simulink model "scattering_based_bi_teleop_pf2"  (R2020b)
settings: Solver=VariableStepAuto  StartTime=0.0  StopTime=4.0  RelTol=1e-3
values from neighbouring files (symbols this model uses):
  A = 1    [four_channel_bilateral_teleoperation_kalman_params.m]    (also in four_channel_bilateral_teleoperation_params.m; kalman_test.m = [1 Ts Ts^2/2; 0 1 Ts; 0 0 1]; recursive_estimation.m = [1 Ts Ts^2/2; 0 1 Ts; 0 0 1]; scattering_based_bi_teleop_pf_kalman_params.m)
  b = 1    [scattering_based_bi_teleop_pf_kalman_params.m]    (also in scattering_based_bi_teleop_pf_params.m; scattering_based_bi_teleop_pp_kalman_params.m; scattering_based_bi_teleop_pp_params.m = 0.9; scattering_based_bilateral_teleoperation_pp_params.m = 0.234)
  Be = 100    [four_channel_bilateral_teleoperation_architecture_params.m]    (also in four_channel_bilateral_teleoperation_kalman_params.m = 0; four_channel_bilateral_teleoperation_params.m = 0; scattering_based_bi_teleop_pf_kalman_params.m = 10; scattering_based_bi_teleop_pf_params.m = 10)
  Bh = 70    [four_channel_bilateral_teleoperation_architecture_params.m]    (also in four_channel_bilateral_teleoperation_kalman_params.m; four_channel_bilateral_teleoperation_params.m; scattering_based_bi_teleop_pf_kalman_params.m = 1.5; scattering_based_bi_teleop_pf_params.m = 1.5)
  Bm = 1    [four_channel_bilateral_teleoperation_architecture_params.m]    (also in four_channel_bilateral_teleoperation_kalman_params.m = 0.8; four_channel_bilateral_teleoperation_params.m = 0.8; scattering_based_bi_teleop_pf_kalman_params.m = 0; scattering_based_bi_teleop_pf_params.m = 0)
  Bs = 1    [four_channel_bilateral_teleoperation_architecture_params.m]    (also in four_channel_bilateral_teleoperation_kalman_params.m = 3.2; four_channel_bilateral_teleoperation_params.m = 3.2; scattering_based_bi_teleop_pf_kalman_params.m = 40; scattering_based_bi_teleop_pf_params.m = 3)
  delay = 10    [scattering_based_bi_teleop_pf_kalman_params.m]    (also in scattering_based_bi_teleop_pf_params.m = 1; scattering_based_bi_teleop_pp_kalman_params.m = 1; scattering_based_bi_teleop_pp_params.m = 1; tank_based_bi_teleop_pf_kalman.m)
  Dh = 500    [four_channel_bilateral_teleoperation_kalman_params.m]    (also in four_channel_bilateral_teleoperation_params.m; scattering_based_bi_teleop_pf_kalman_params.m = 0; scattering_based_bi_teleop_pf_params.m = 17; scattering_based_bi_teleop_pp_kalman_params.m = 0)
  Dm = 5    [four_channel_bilateral_teleoperation_architecture_params.m]    (also in four_channel_bilateral_teleoperation_kalman_params.m = 0; four_channel_bilateral_teleoperation_params.m = 0; scattering_based_bi_teleop_pf_kalman_params.m = 0; scattering_based_bi_teleop_pf_params.m = 0)
  Ds = 10    [four_channel_bilateral_teleoperation_architecture_params.m]    (also in four_channel_bilateral_teleoperation_kalman_params.m = 0; four_channel_bilateral_teleoperation_params.m = 0; scattering_based_bi_teleop_pf_kalman_params.m = 0; scattering_based_bi_teleop_pf_params.m = 0)
  Fc = 1    [four_channel_bilateral_teleoperation_kalman_params.m]    (also in four_channel_bilateral_teleoperation_params.m; kalman_test.m = 10; scattering_based_bi_teleop_pf_kalman_params.m = 0.1; scattering_based_bi_teleop_pf_params.m)
  Filter = 8    [scattering_based_bi_teleop_pf_kalman_params.m]    (also in scattering_based_bi_teleop_pf_params.m = 100; scattering_based_bi_teleop_pp_kalman_params.m = 10; scattering_based_bi_teleop_pp_params.m = 5; tank_based_bi_teleop_pf_kalman.m = 100)
  Fip = 1    [four_channel_bilateral_teleoperation_kalman_params.m]    (also in four_channel_bilateral_teleoperation_params.m; scattering_based_bi_teleop_pf_kalman_params.m = 5; scattering_based_bi_teleop_pf_params.m = 10; scattering_based_bi_teleop_pp_kalman_params.m = 5)
  Je = 0    [four_channel_bilateral_teleoperation_architecture_params.m]    (also in four_channel_bilateral_teleoperation_kalman_params.m; four_channel_bilateral_teleoperation_params.m; scattering_based_bi_teleop_pf_kalman_params.m; scattering_based_bi_teleop_pf_params.m)
  Jh = 0.5    [four_channel_bilateral_teleoperation_architecture_params.m]    (also in four_channel_bilateral_teleoperation_kalman_params.m; four_channel_bilateral_teleoperation_params.m; scattering_based_bi_teleop_pf_kalman_params.m = 0; scattering_based_bi_teleop_pf_params.m = 0.05)
  Ke = 200    [four_channel_bilateral_teleoperation_architecture_params.m]    (also in four_channel_bilateral_teleoperation_kalman_params.m = 50; four_channel_bilateral_teleoperation_params.m = 50; scattering_based_bi_teleop_pf_kalman_params.m; scattering_based_bi_teleop_pf_params.m)
  Kh = 2000    [four_channel_bilateral_teleoperation_architecture_params.m]    (also in four_channel_bilateral_teleoperation_kalman_params.m; four_channel_bilateral_teleoperation_params.m; scattering_based_bi_teleop_pf_kalman_params.m = 1; scattering_based_bi_teleop_pf_params.m = 0)
  Km = 1    [four_channel_bilateral_teleoperation_architecture_params.m]    (also in four_channel_bilateral_teleoperation_kalman_params.m; four_channel_bilateral_teleoperation_params.m; scattering_based_bi_teleop_pf_kalman_params.m = 0; scattering_based_bi_teleop_pf_params.m = 0)
  Ks = 1    [four_channel_bilateral_teleoperation_architecture_params.m]    (also in four_channel_bilateral_teleoperation_kalman_params.m = 4; four_channel_bilateral_teleoperation_params.m = 4; scattering_based_bi_teleop_pf_kalman_params.m = 50; scattering_based_bi_teleop_pf_params.m = 110)
  Mm = 0.5    [four_channel_bilateral_teleoperation_architecture_params.m]    (also in four_channel_bilateral_teleoperation_kalman_params.m; four_channel_bilateral_teleoperation_params.m; scattering_based_bi_teleop_pf_kalman_params.m; scattering_based_bi_teleop_pf_params.m)
  Ms = 2    [four_channel_bilateral_teleoperation_architecture_params.m]    (also in four_channel_bilateral_teleoperation_kalman_params.m; four_channel_bilateral_teleoperation_params.m; scattering_based_bi_teleop_pf_kalman_params.m; scattering_based_bi_teleop_pf_params.m)
  Ph = 2000    [four_channel_bilateral_teleoperation_kalman_params.m]    (also in four_channel_bilateral_teleoperation_params.m = 50500; scattering_based_bi_teleop_pf_kalman_params.m = 5; scattering_based_bi_teleop_pf_params.m = 23; scattering_based_bi_teleop_pp_kalman_params.m = 6)
  Ts = 0.001    [four_channel_bilateral_teleoperation_kalman_params.m]    (also in four_channel_bilateral_teleoperation_params.m; kalman_test.m; recursive_estimation.m; scattering_based_bi_teleop_pf_kalman_params.m)
settings Model: Creator=anuj  LastModifiedBy=filippo

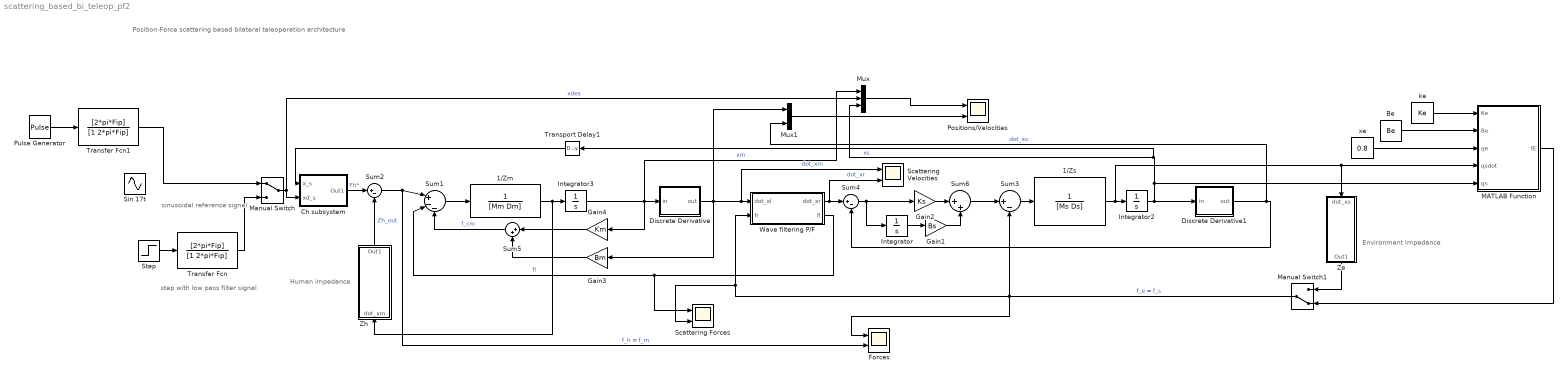
== system scattering_based_bi_teleop_pf2 ==
  note: Position-Force scattering based bilateral teleoperation architecture
  note: Environment Impedance
  note: Human impedance
  note: sinusoidal reference signal
  note: step with low pass filter signal
  1/Zm : TransferFcn  Denominator=[Mm Dm]
  1/Zs : TransferFcn  Denominator=[Ms Ds]
  Be : Constant  Value=Be
  Ch subsystem : Subsystem
  Discrete Derivative : Subsystem
  Discrete Derivative1 : Subsystem
  Forces : Scope  NumInputPorts=2
  Gain1 : Gain  Gain=Bs
  Gain2 : Gain  Gain=Ks
  Gain3 : Gain  Gain=Bm
  Gain4 : Gain  Gain=Km
  Integrator : Integrator
  Integrator2 : Integrator
  Integrator3 : Integrator
  MATLAB Function : MATLAB Function  TreatAsAtomicUnit=on
  Manual Switch : ManualSwitch
  Manual Switch1 : ManualSwitch  CurrentSetting=0
  Mux : Mux  Inputs=3
  Mux1 : Mux  Inputs=2
  Positions/Velocities : Scope  NumInputPorts=2
  Pulse Generator : DiscretePulseGenerator  PulseType=Time based  Amplitude=A  PulseWidth=50  PhaseDelay=1
  Scattering Forces : Scope  NumInputPorts=2
  Scattering Velocities : Scope  NumInputPorts=2
  Sin 17t : Sin  Amplitude=A  Frequency=2*pi*Fc  SampleTime=0
  Step : Step  After=A  SampleTime=0
  Sum1 : Sum  Inputs=|+--
  Sum2 : Sum  Inputs=|+-
  Sum3 : Sum  Inputs=|+-
  Sum4 : Sum  Inputs=|+-
  Sum5 : Sum  Inputs=|++
  Sum6 : Sum  Inputs=|++
  Transfer Fcn : TransferFcn  Numerator=[2*pi*Fip]  Denominator=[1 2*pi*Fip]
  Transfer Fcn1 : TransferFcn  Numerator=[2*pi*Fip]  Denominator=[1 2*pi*Fip]
  Transport Delay1 : TransportDelay  DelayTime=delay*Ts
  Wave filtering P/F : Subsystem
  Ze : Subsystem
  Zh : Subsystem
  ke : Constant  Value=Ke
  xe : Constant  Value=0.8
  wires:
  Sum2/1 -> Forces/2, Sum1/1  "f_h = f_m"
  1/Zm/1 -> Integrator3/1, Zh/1(dot_xm)
  Sum1/1 -> 1/Zm/1
  Wave filtering P/F/2(fl) -> Sum1/2, Scattering Forces/1  "fl"
  Sum3/1 -> 1/Zs/1
  Manual Switch1/1 -> Wave filtering P/F/2(fr), Scattering Forces/2, Forces/1, Sum3/2  "f_e = f_s"
  Be/1 -> MATLAB Function/2(Be)
  xe/1 -> MATLAB Function/3(qe)
  ke/1 -> MATLAB Function/1(Ke)
  Transfer Fcn/1 -> Manual Switch/2
  Step/1 -> Transfer Fcn/1
  Zh/1(Out1) -> Sum2/2  "Zh_out"
  Discrete Derivative1/1(out) -> Sum4/2, Mux1/2  "dot_xs"
  1/Zs/1 -> Integrator2/1, Ze/1(dot_xs), MATLAB Function/4(qsdot)
  Integrator2/1 -> Discrete Derivative1/1(in), Transport Delay1/1, Mux/3, MATLAB Function/5(qs)  "xs"
  Integrator3/1 -> Mux/1, Gain4/1, Discrete Derivative/1(in)  "xm"
  Discrete Derivative/1(out) -> Gain3/1, Mux1/1, Scattering Velocities/1, Wave filtering P/F/1(dot_xl)  "dot_xm"
  Ze/1(Out1) -> Manual Switch1/1
  MATLAB Function/1(fE) -> Manual Switch1/2
  Mux1/1 -> Positions/Velocities/2
  Mux/1 -> Positions/Velocities/1
  Manual Switch/1 -> Mux/2, Ch subsystem/2(xd_s)  "xdes"
  Ch subsystem/1(Out1) -> Sum2/1  "Fh*"
  Sum6/1 -> Sum3/1
  Gain1/1 -> Sum6/2
  Gain2/1 -> Sum6/1
  Integrator/1 -> Gain1/1
  Wave filtering P/F/1(dot_xr) -> Sum4/1, Scattering Velocities/2  "dot_xr"
  Sum4/1 -> Integrator/1, Gain2/1
  Gain4/1 -> Sum5/1
  Sum5/1 -> Sum1/3  "f_cm"
  Gain3/1 -> Sum5/2
  Pulse Generator/1 -> Transfer Fcn1/1
  Transfer Fcn1/1 -> Manual Switch/1
  Transport Delay1/1 -> Ch subsystem/1(x_s)

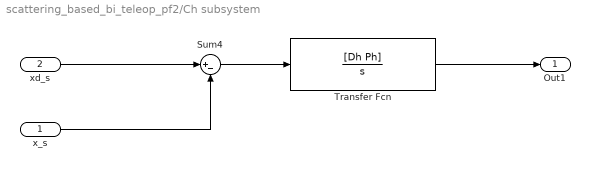
== system scattering_based_bi_teleop_pf2/Ch subsystem ==
  x_s : Inport
  xd_s : Inport  Port=2
  Sum4 : Sum  Inputs=|+-
  Transfer Fcn : TransferFcn  Numerator=[Dh Ph]  Denominator=[1 0]
  Out1 : Outport
  wires:
  xd_s/1 -> Sum4/1
  Sum4/1 -> Transfer Fcn/1
  Transfer Fcn/1 -> Out1/1
  x_s/1 -> Sum4/2

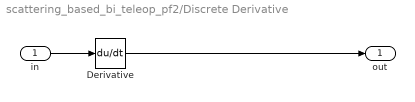
== system scattering_based_bi_teleop_pf2/Discrete Derivative ==
  in : Inport
  Derivative : Derivative
  out : Outport
  wires:
  in/1 -> Derivative/1
  Derivative/1 -> out/1

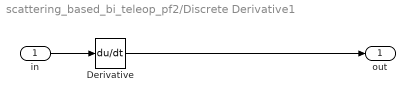
== system scattering_based_bi_teleop_pf2/Discrete Derivative1 ==
  in : Inport
  Derivative : Derivative
  out : Outport
  wires:
  in/1 -> Derivative/1
  Derivative/1 -> out/1

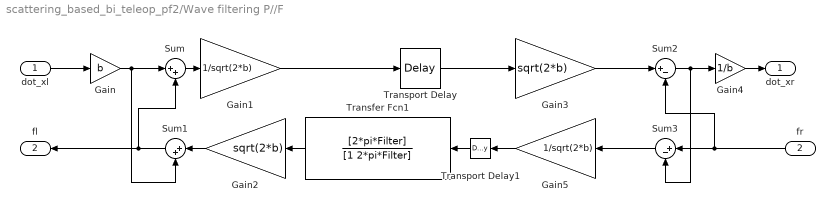
== system scattering_based_bi_teleop_pf2/Wave filtering P//F ==
  dot_xl : Inport
  fr : Inport  Port=2
  Gain : Gain  Gain=b
  Gain1 : Gain  Gain=1/sqrt(2*b)
  Gain2 : Gain  Gain=sqrt(2*b)
  Gain3 : Gain  Gain=sqrt(2*b)
  Gain4 : Gain  Gain=1/b
  Gain5 : Gain  Gain=1/sqrt(2*b)
  Sum : Sum  Inputs=|++
  Sum1 : Sum  Inputs=|++
  Sum2 : Sum  Inputs=|+-
  Sum3 : Sum  Inputs=|+-
  Transfer Fcn1 : TransferFcn  Numerator=[2*pi*Filter]  Denominator=[1 2*pi*Filter]
  Transport Delay : TransportDelay  DelayTime=delay*Ts
  Transport Delay1 : TransportDelay  DelayTime=delay*Ts
  dot_xr : Outport
  fl : Outport  Port=2
  wires:
  Sum2/1 -> Sum3/2, Gain4/1
  Gain/1 -> Sum1/2, Sum/1
  Sum/1 -> Gain1/1
  Gain2/1 -> Sum1/1
  fr/1 -> Sum2/2, Sum3/1
  Sum3/1 -> Gain5/1
  Gain3/1 -> Sum2/1
  Transport Delay/1 -> Gain3/1
  dot_xl/1 -> Gain/1
  Gain4/1 -> dot_xr/1
  Sum1/1 -> fl/1, Sum/2
  Transfer Fcn1/1 -> Gain2/1
  Gain5/1 -> Transport Delay1/1
  Transport Delay1/1 -> Transfer Fcn1/1
  Gain1/1 -> Transport Delay/1

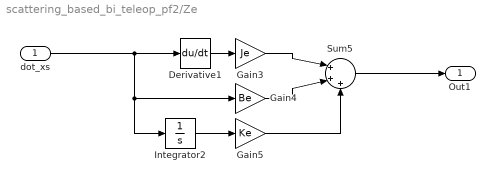
== system scattering_based_bi_teleop_pf2/Ze ==
  dot_xs : Inport
  Derivative1 : Derivative
  Gain3 : Gain  Gain=Je
  Gain4 : Gain  Gain=Be
  Gain5 : Gain  Gain=Ke
  Integrator2 : Integrator
  Sum5 : Sum  Inputs=|+++
  Out1 : Outport
  wires:
  Gain4/1 -> Sum5/2
  Gain3/1 -> Sum5/1
  Gain5/1 -> Sum5/3
  Sum5/1 -> Out1/1
  Integrator2/1 -> Gain5/1
  dot_xs/1 -> Integrator2/1, Gain4/1, Derivative1/1
  Derivative1/1 -> Gain3/1

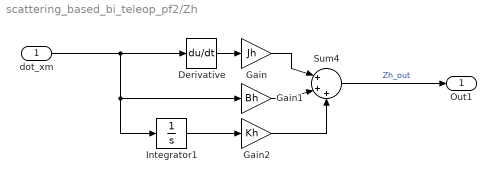
== system scattering_based_bi_teleop_pf2/Zh ==
  dot_xm : Inport
  Derivative : Derivative
  Gain : Gain  Gain=Jh
  Gain1 : Gain  Gain=Bh
  Gain2 : Gain  Gain=Kh
  Integrator1 : Integrator
  Sum4 : Sum  Inputs=|+++
  Out1 : Outport
  wires:
  Derivative/1 -> Gain/1
  Integrator1/1 -> Gain2/1
  Gain2/1 -> Sum4/3
  Gain1/1 -> Sum4/2
  Gain/1 -> Sum4/1
  Sum4/1 -> Out1/1  "Zh_out"
  dot_xm/1 -> Gain1/1, Integrator1/1, Derivative/1

== matlab function scattering_based_bi_teleop_pf2/MATLAB Function ==
  data: Ke input; fE output; Be input; qe input; qsdot input; qs input
function fE = environment(Ke, Be, qe, qsdot, qs)
    if qs > qe
        fE = Ke * (qs - qe) + Be * qsdot; % Plot both contributions Ke and Be
    else
        fE = 0;
    end
end
